simulink model "PendulumModel"  (R2020a)
settings: Solver=VariableStepAuto  StartTime=0.0  StopTime=10.0  RelTol=1e-3
values from neighbouring files (symbols this model uses):
  A = [0 1          0                0 ... (first row only)    [ModelParameters.m]
  B = [0; 1/M; 0; s*1/(M*L)]    [ModelParameters.m]
  y0 = [0; 0; pi+.0001; 0]    [ModelParameters.m]
libraries: rllib x1, simulink x1
settings Model: Creator=A Weirdo  LastModifiedBy=A Weirdo

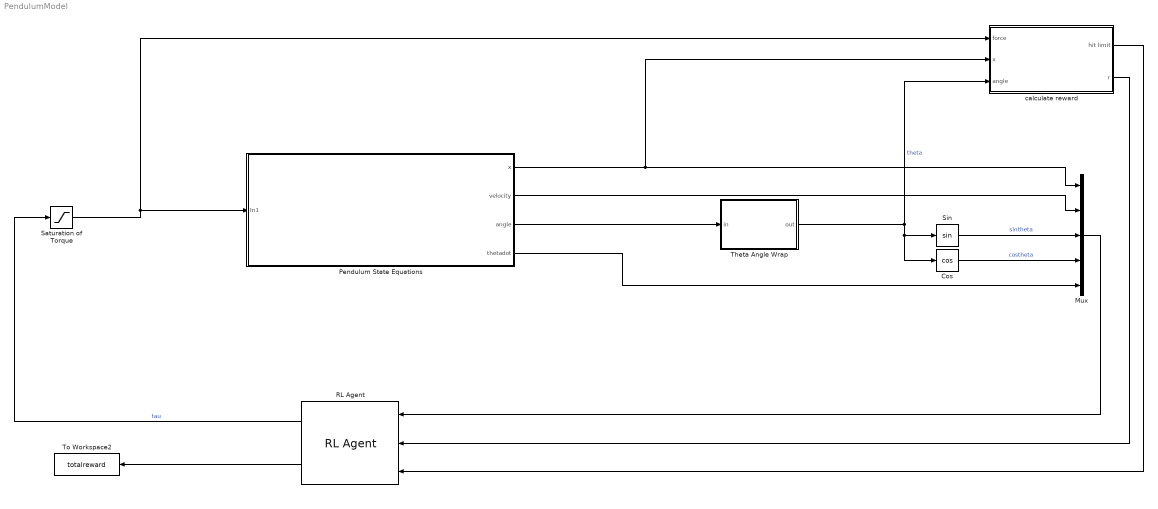
== system PendulumModel ==
  Cos : Trigonometry  Operator=cos
  Mux : Mux  Inputs=5
  Pendulum State Equations : Subsystem
  RL Agent : rllib/RL Agent  Agent=agent  ProvideReward=on  ProvideIsDone=on  ProvideCumRwd=on  TreatAsDirectFeedthrough=on  CollectLoggedSignals=on  CollectModelStates=on
  Saturation of Torque : Saturate  UpperLimit=10  LowerLimit=-10
  Sin : Trigonometry  OutputSignalType=real
  "Theta Angle Wrap " : Subsystem
  To Workspace2 : ToWorkspace  VariableName=totalreward  SaveFormat=Timeseries  SampleTime=-1
  calculate reward : Subsystem
  wires:
  calculate reward/2(r) -> RL Agent/2
  calculate reward/1(hit limit) -> RL Agent/3
  "Theta Angle Wrap "/1(out) -> Cos/1, Sin/1, calculate reward/3(angle)  "theta"
  RL Agent/2 -> To Workspace2/1
  Saturation of Torque/1 -> Pendulum State Equations/1(In1), calculate reward/1(force)
  Pendulum State Equations/1(x) -> Mux/1, calculate reward/2(x)
  Pendulum State Equations/3(angle) -> "Theta Angle Wrap "/1(in)
  Pendulum State Equations/4(thetadot) -> Mux/5
  Cos/1 -> Mux/4  "costheta"
  Sin/1 -> Mux/3  "sintheta"
  Pendulum State Equations/2(velocity) -> Mux/2
  RL Agent/1 -> Saturation of Torque/1  "tau"
  Mux/1 -> RL Agent/1

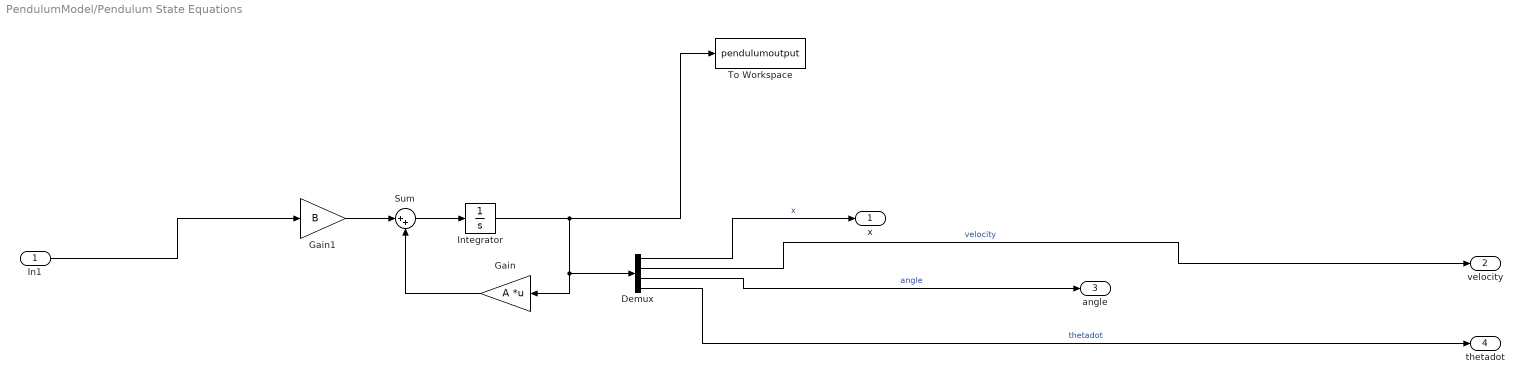
== system PendulumModel/Pendulum State Equations ==
  In1 : Inport
  Demux : Demux
  Gain : Gain  Gain=A  Multiplication=Matrix(K*u) (u vector)
  Gain1 : Gain  Gain=B
  Integrator : Integrator  InitialCondition=y0
  Sum : Sum  Inputs=|++
  To Workspace : ToWorkspace  VariableName=pendulumoutput  SaveFormat=Timeseries  SampleTime=-1
  x : Outport
  velocity : Outport  Port=2
  angle : Outport  Port=3
  thetadot : Outport  Port=4
  wires:
  Demux/4 -> thetadot/1  "thetadot"
  Sum/1 -> Integrator/1
  Demux/1 -> x/1  "x"
  Demux/2 -> velocity/1  "velocity"
  Gain1/1 -> Sum/1
  Demux/3 -> angle/1  "angle"
  In1/1 -> Gain1/1
  Integrator/1 -> To Workspace/1, Gain/1, Demux/1
  Gain/1 -> Sum/2

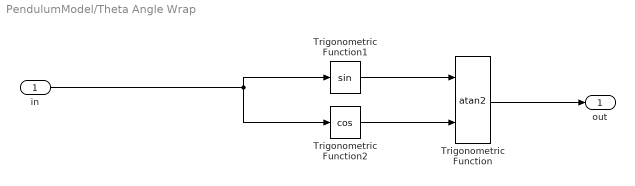
== system PendulumModel/Theta Angle Wrap  ==
  in : Inport
  Trigonometric Function : Trigonometry  Operator=atan2  OutputSignalType=real
  Trigonometric Function1 : Trigonometry
  Trigonometric Function2 : Trigonometry  Operator=cos
  out : Outport
  wires:
  in/1 -> Trigonometric Function1/1, Trigonometric Function2/1
  Trigonometric Function1/1 -> Trigonometric Function/1
  Trigonometric Function2/1 -> Trigonometric Function/2
  Trigonometric Function/1 -> out/1

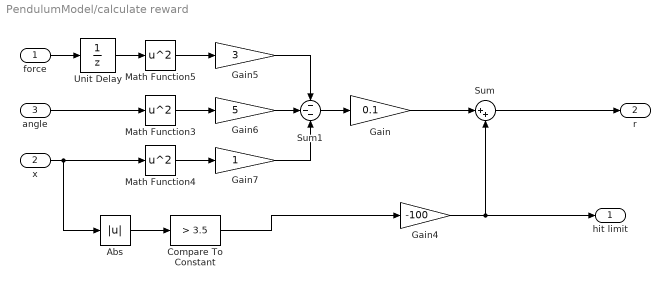
== system PendulumModel/calculate reward ==
  force : Inport
  x : Inport  Port=2
  angle : Inport  Port=3
  Abs : Abs
  Compare To Constant : simulink/Logic and Bit Operations/Compare To Constant  relop=>  const=3.5  OutDataTypeStr=boolean
  Gain : Gain  Gain=0.1
  Gain4 : Gain  Gain=-100
  Gain5 : Gain  Gain=3
  Gain6 : Gain  Gain=5
  Gain7 : Gain
  Math Function3 : Math  Operator=square  SignedPower=on  SaturateOnIntegerOverflow=on
  Math Function4 : Math  Operator=square  SignedPower=on  SaturateOnIntegerOverflow=on
  Math Function5 : Math  Operator=square  SignedPower=on  SaturateOnIntegerOverflow=on
  Sum : Sum  Inputs=|++
  Sum1 : Sum  Inputs=---
  Unit Delay : UnitDelay  SampleTime=-1  HasFrameUpgradeWarning=on
  hit limit : Outport  VectorParamsAs1DForOutWhenUnconnected=off
  r : Outport  Port=2  VectorParamsAs1DForOutWhenUnconnected=off
  wires:
  Compare To Constant/1 -> Gain4/1
  Abs/1 -> Compare To Constant/1
  Gain5/1 -> Sum1/1
  Gain6/1 -> Sum1/2
  x/1 -> Abs/1, Math Function4/1
  Sum1/1 -> Gain/1
  Math Function3/1 -> Gain6/1
  Math Function5/1 -> Gain5/1
  Gain7/1 -> Sum1/3
  Math Function4/1 -> Gain7/1
  force/1 -> Unit Delay/1
  Unit Delay/1 -> Math Function5/1
  Sum/1 -> r/1
  angle/1 -> Math Function3/1
  Gain/1 -> Sum/1
  Gain4/1 -> hit limit/1, Sum/2
